simulink library "speedgoatlib_mscp"  (R2024b)
settings: Solver=VariableStepAuto  StartTime=0.0  StopTime=10.0  RelTol=1e-3
libraries: slrealtimeethercatlib x517, simulink x316, hdlsllib x168, $bdroot x11, slrealtimeutilitieslib x1
(part 2 of 5)

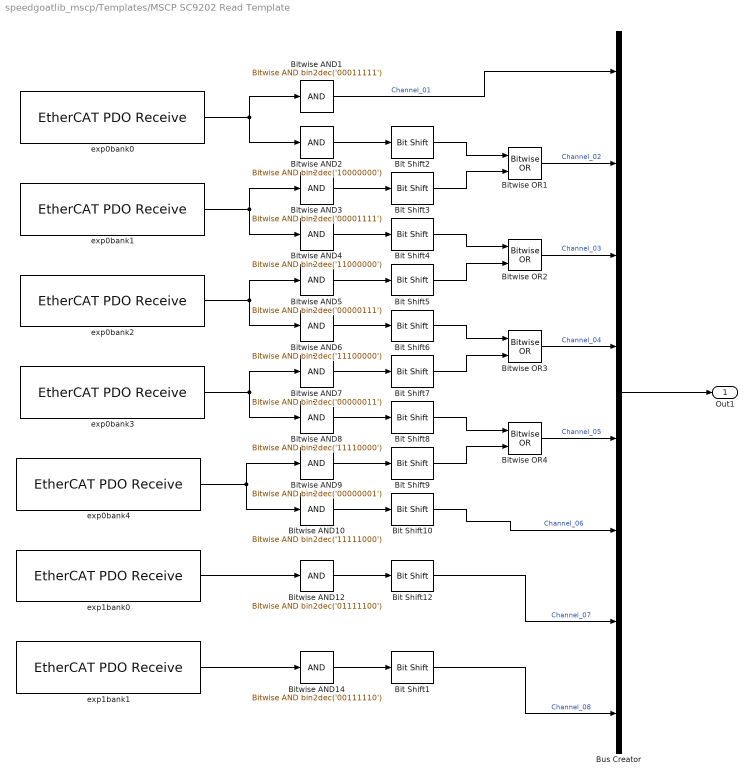
== system speedgoatlib_mscp/Templates/MSCP SC9202 Read Template ==
  Bit Shift1 : hdlsllib/Logic and Bit Operations/Bit Shift  mode=Shift Right Logical  N=1
  Bit Shift10 : hdlsllib/Logic and Bit Operations/Bit Shift  mode=Shift Right Logical  N=3
  Bit Shift12 : hdlsllib/Logic and Bit Operations/Bit Shift  mode=Shift Right Logical  N=2
  Bit Shift2 : hdlsllib/Logic and Bit Operations/Bit Shift  mode=Shift Right Logical  N=7
  Bit Shift3 : hdlsllib/Logic and Bit Operations/Bit Shift  mode=Shift Left Logical  N=1
  Bit Shift4 : hdlsllib/Logic and Bit Operations/Bit Shift  mode=Shift Right Logical  N=6
  Bit Shift5 : hdlsllib/Logic and Bit Operations/Bit Shift  mode=Shift Left Logical  N=2
  Bit Shift6 : hdlsllib/Logic and Bit Operations/Bit Shift  mode=Shift Right Logical  N=5
  Bit Shift7 : hdlsllib/Logic and Bit Operations/Bit Shift  mode=Shift Left Logical  N=3
  Bit Shift8 : hdlsllib/Logic and Bit Operations/Bit Shift  mode=Shift Right Logical  N=4
  Bit Shift9 : hdlsllib/Logic and Bit Operations/Bit Shift  mode=Shift Left Logical  N=4
  Bitwise AND1 : simulink/Logic and Bit Operations/Bitwise Operator  logicop=AND  UseBitMask=on  BitMask=bin2dec('00011111')  BitMaskRealWorld=Stored Integer
      settings: LibrarySourceBlock=|
      | simulink/Quick Insert/Logic and Bit
      | Operations/Bitwise AND
  Bitwise AND10 : simulink/Logic and Bit Operations/Bitwise Operator  logicop=AND  UseBitMask=on  BitMask=bin2dec('11111000')  BitMaskRealWorld=Stored Integer
      settings: LibrarySourceBlock=|
      | simulink/Quick Insert/Logic and Bit
      | Operations/Bitwise AND
  Bitwise AND12 : simulink/Logic and Bit Operations/Bitwise Operator  logicop=AND  UseBitMask=on  BitMask=bin2dec('01111100')  BitMaskRealWorld=Stored Integer
      settings: LibrarySourceBlock=|
      | simulink/Quick Insert/Logic and Bit
      | Operations/Bitwise AND
  Bitwise AND14 : simulink/Logic and Bit Operations/Bitwise Operator  logicop=AND  UseBitMask=on  BitMask=bin2dec('00111110')  BitMaskRealWorld=Stored Integer
      settings: LibrarySourceBlock=|
      | simulink/Quick Insert/Logic and Bit
      | Operations/Bitwise AND
  Bitwise AND2 : simulink/Logic and Bit Operations/Bitwise Operator  logicop=AND  UseBitMask=on  BitMask=bin2dec('10000000')  BitMaskRealWorld=Stored Integer
      settings: LibrarySourceBlock=|
      | simulink/Quick Insert/Logic and Bit
      | Operations/Bitwise AND
  Bitwise AND3 : simulink/Logic and Bit Operations/Bitwise Operator  logicop=AND  UseBitMask=on  BitMask=bin2dec('00001111')  BitMaskRealWorld=Stored Integer
      settings: LibrarySourceBlock=|
      | simulink/Quick Insert/Logic and Bit
      | Operations/Bitwise AND
  Bitwise AND4 : simulink/Logic and Bit Operations/Bitwise Operator  logicop=AND  UseBitMask=on  BitMask=bin2dec('11000000')  BitMaskRealWorld=Stored Integer
      settings: LibrarySourceBlock=|
      | simulink/Quick Insert/Logic and Bit
      | Operations/Bitwise AND
  Bitwise AND5 : simulink/Logic and Bit Operations/Bitwise Operator  logicop=AND  UseBitMask=on  BitMask=bin2dec('00000111')  BitMaskRealWorld=Stored Integer
      settings: LibrarySourceBlock=|
      | simulink/Quick Insert/Logic and Bit
      | Operations/Bitwise AND
  Bitwise AND6 : simulink/Logic and Bit Operations/Bitwise Operator  logicop=AND  UseBitMask=on  BitMask=bin2dec('11100000')  BitMaskRealWorld=Stored Integer
      settings: LibrarySourceBlock=|
      | simulink/Quick Insert/Logic and Bit
      | Operations/Bitwise AND
  Bitwise AND7 : simulink/Logic and Bit Operations/Bitwise Operator  logicop=AND  UseBitMask=on  BitMask=bin2dec('00000011')  BitMaskRealWorld=Stored Integer
      settings: LibrarySourceBlock=|
      | simulink/Quick Insert/Logic and Bit
      | Operations/Bitwise AND
  Bitwise AND8 : simulink/Logic and Bit Operations/Bitwise Operator  logicop=AND  UseBitMask=on  BitMask=bin2dec('11110000')  BitMaskRealWorld=Stored Integer
      settings: LibrarySourceBlock=|
      | simulink/Quick Insert/Logic and Bit
      | Operations/Bitwise AND
  Bitwise AND9 : simulink/Logic and Bit Operations/Bitwise Operator  logicop=AND  UseBitMask=on  BitMask=bin2dec('00000001')  BitMaskRealWorld=Stored Integer
      settings: LibrarySourceBlock=|
      | simulink/Quick Insert/Logic and Bit
      | Operations/Bitwise AND
  Bitwise OR{1..4} (4 alike) : simulink/Logic and Bit Operations/Bitwise Operator  logicop=OR  UseBitMask=off  NumInputPorts=2  BitMask=bin2dec('11011001')  BitMaskRealWorld=Stored Integer
      settings: LibrarySourceBlock=|
      | simulink/Quick Insert/Logic and Bit
      | Operations/Bitwise OR
  Bus Creator : BusCreator  Inputs=8  OutDataTypeStr=Bus: MscpBus_SC9202
      settings: InheritFromInputs=off
  exp0bank{0..4} (5 alike) : slrealtimeethercatlib/EtherCAT PDO Receive  Priority=2  sig_name=Uninitialized Block  sig_offset=144  sig_type=uint8  type_size=8  sig_dim=1  device_id=0  sample_time=0.010000
  exp1bank0 : slrealtimeethercatlib/EtherCAT PDO Receive  Priority=2  sig_name=Uninitialized Block  sig_offset=144  sig_type=uint8  type_size=8  sig_dim=1  device_id=0  sample_time=0.010000
  exp1bank1 : slrealtimeethercatlib/EtherCAT PDO Receive  Priority=2  sig_name=Uninitialized Block  sig_offset=144  sig_type=uint8  type_size=8  sig_dim=1  device_id=0  sample_time=0.010000
  Out1 : Outport
  wires:
  Bit Shift1/1 -> Bus Creator/8  "Channel_08"
  Bitwise AND14/1 -> Bit Shift1/1
  Bit Shift5/1 -> Bitwise OR2/2
  exp0bank3/1 -> Bitwise AND8/1, Bitwise AND7/1
  Bitwise OR2/1 -> Bus Creator/3  "Channel_03"
  exp1bank1/1 -> Bitwise AND14/1
  exp0bank4/1 -> Bitwise AND10/1, Bitwise AND9/1
  exp0bank0/1 -> Bitwise AND2/1, Bitwise AND1/1
  exp1bank0/1 -> Bitwise AND12/1
  exp0bank1/1 -> Bitwise AND3/1, Bitwise AND4/1
  Bitwise OR4/1 -> Bus Creator/5  "Channel_05"
  Bitwise AND8/1 -> Bit Shift8/1
  Bit Shift3/1 -> Bitwise OR1/2
  Bitwise AND12/1 -> Bit Shift12/1
  Bit Shift7/1 -> Bitwise OR3/2
  Bitwise AND6/1 -> Bit Shift6/1
  Bitwise OR1/1 -> Bus Creator/2  "Channel_02"
  exp0bank2/1 -> Bitwise AND5/1, Bitwise AND6/1
  Bit Shift8/1 -> Bitwise OR4/1
  Bit Shift12/1 -> Bus Creator/7  "Channel_07"
  Bit Shift9/1 -> Bitwise OR4/2
  Bit Shift2/1 -> Bitwise OR1/1
  Bitwise AND10/1 -> Bit Shift10/1
  Bitwise AND1/1 -> Bus Creator/1  "Channel_01"
  Bit Shift6/1 -> Bitwise OR3/1
  Bitwise AND4/1 -> Bit Shift4/1
  Bitwise OR3/1 -> Bus Creator/4  "Channel_04"
  Bit Shift10/1 -> Bus Creator/6  "Channel_06"
  Bus Creator/1 -> Out1/1
  Bitwise AND7/1 -> Bit Shift7/1
  Bitwise AND5/1 -> Bit Shift5/1
  Bitwise AND9/1 -> Bit Shift9/1
  Bitwise AND2/1 -> Bit Shift2/1
  Bit Shift4/1 -> Bitwise OR2/1
  Bitwise AND3/1 -> Bit Shift3/1

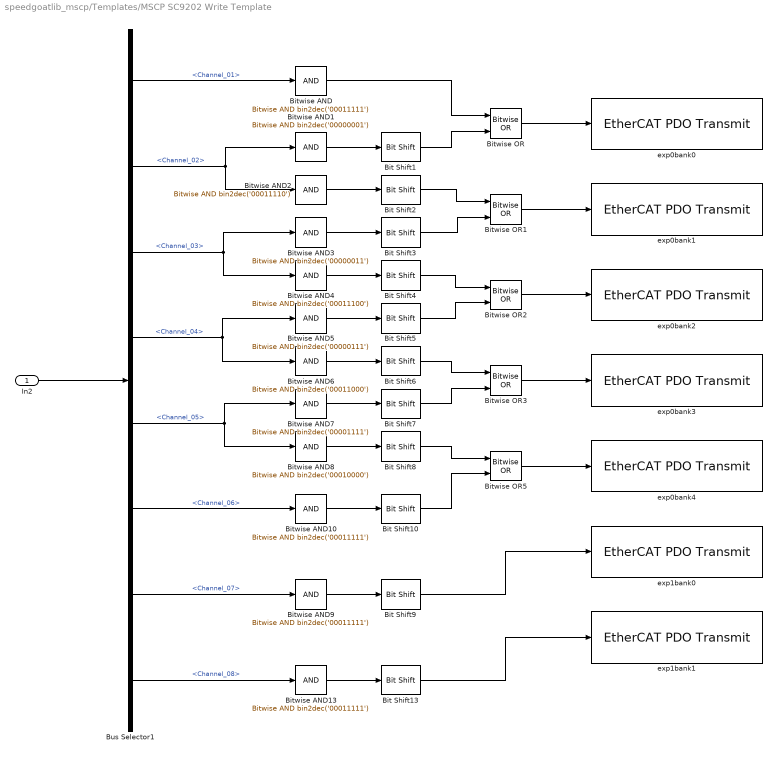
== system speedgoatlib_mscp/Templates/MSCP SC9202 Write Template ==
  In2 : Inport  OutDataTypeStr=Bus: MscpBus_SC9202
  Bit Shift1 : hdlsllib/Logic and Bit Operations/Bit Shift  mode=Shift Left Logical  N=7
  Bit Shift10 : hdlsllib/Logic and Bit Operations/Bit Shift  mode=Shift Left Logical  N=3
  Bit Shift13 : hdlsllib/Logic and Bit Operations/Bit Shift  mode=Shift Left Logical  N=1
  Bit Shift2 : hdlsllib/Logic and Bit Operations/Bit Shift  mode=Shift Right Logical  N=1
  Bit Shift3 : hdlsllib/Logic and Bit Operations/Bit Shift  mode=Shift Left Logical  N=6
  Bit Shift4 : hdlsllib/Logic and Bit Operations/Bit Shift  mode=Shift Right Logical  N=2
  Bit Shift5 : hdlsllib/Logic and Bit Operations/Bit Shift  mode=Shift Left Logical  N=5
  Bit Shift6 : hdlsllib/Logic and Bit Operations/Bit Shift  mode=Shift Right Logical  N=3
  Bit Shift7 : hdlsllib/Logic and Bit Operations/Bit Shift  mode=Shift Left Logical  N=4
  Bit Shift8 : hdlsllib/Logic and Bit Operations/Bit Shift  mode=Shift Right Logical  N=4
  Bit Shift9 : hdlsllib/Logic and Bit Operations/Bit Shift  mode=Shift Left Logical  N=2
  Bitwise AND{,9..10,13} (4 alike) : simulink/Logic and Bit Operations/Bitwise Operator  logicop=AND  UseBitMask=on  BitMask=bin2dec('00011111')  BitMaskRealWorld=Stored Integer
      settings: LibrarySourceBlock=|
      | simulink/Quick Insert/Logic and Bit
      | Operations/Bitwise AND
  Bitwise AND1 : simulink/Logic and Bit Operations/Bitwise Operator  logicop=AND  UseBitMask=on  BitMask=bin2dec('00000001')  BitMaskRealWorld=Stored Integer
      settings: LibrarySourceBlock=|
      | simulink/Quick Insert/Logic and Bit
      | Operations/Bitwise AND
  Bitwise AND2 : simulink/Logic and Bit Operations/Bitwise Operator  logicop=AND  UseBitMask=on  BitMask=bin2dec('00011110')  BitMaskRealWorld=Stored Integer
      settings: LibrarySourceBlock=|
      | simulink/Quick Insert/Logic and Bit
      | Operations/Bitwise AND
  Bitwise AND3 : simulink/Logic and Bit Operations/Bitwise Operator  logicop=AND  UseBitMask=on  BitMask=bin2dec('00000011')  BitMaskRealWorld=Stored Integer
      settings: LibrarySourceBlock=|
      | simulink/Quick Insert/Logic and Bit
      | Operations/Bitwise AND
  Bitwise AND4 : simulink/Logic and Bit Operations/Bitwise Operator  logicop=AND  UseBitMask=on  BitMask=bin2dec('00011100')  BitMaskRealWorld=Stored Integer
      settings: LibrarySourceBlock=|
      | simulink/Quick Insert/Logic and Bit
      | Operations/Bitwise AND
  Bitwise AND5 : simulink/Logic and Bit Operations/Bitwise Operator  logicop=AND  UseBitMask=on  BitMask=bin2dec('00000111')  BitMaskRealWorld=Stored Integer
      settings: LibrarySourceBlock=|
      | simulink/Quick Insert/Logic and Bit
      | Operations/Bitwise AND
  Bitwise AND6 : simulink/Logic and Bit Operations/Bitwise Operator  logicop=AND  UseBitMask=on  BitMask=bin2dec('00011000')  BitMaskRealWorld=Stored Integer
      settings: LibrarySourceBlock=|
      | simulink/Quick Insert/Logic and Bit
      | Operations/Bitwise AND
  Bitwise AND7 : simulink/Logic and Bit Operations/Bitwise Operator  logicop=AND  UseBitMask=on  BitMask=bin2dec('00001111')  BitMaskRealWorld=Stored Integer
      settings: LibrarySourceBlock=|
      | simulink/Quick Insert/Logic and Bit
      | Operations/Bitwise AND
  Bitwise AND8 : simulink/Logic and Bit Operations/Bitwise Operator  logicop=AND  UseBitMask=on  BitMask=bin2dec('00010000')  BitMaskRealWorld=Stored Integer
      settings: LibrarySourceBlock=|
      | simulink/Quick Insert/Logic and Bit
      | Operations/Bitwise AND
  Bitwise OR{,1..3,5} (5 alike) : simulink/Logic and Bit Operations/Bitwise Operator  logicop=OR  UseBitMask=off  NumInputPorts=2  BitMask=bin2dec('11011001')  BitMaskRealWorld=Stored Integer
      settings: LibrarySourceBlock=|
      | simulink/Quick Insert/Logic and Bit
      | Operations/Bitwise OR
  Bus Selector1 : BusSelector  OutputSignals=Channel_01,Channel_02,Channel_03,Channel_04,Channel_05,Channel_06,Channel_07,Channel_08
  exp0bank{0..4} (5 alike) : slrealtimeethercatlib/EtherCAT PDO Transmit  Priority=3  sig_name=Uninitialized Block  sig_offset=128  sig_type=uint8  type_size=8  sig_dim=1  device_id=0  sample_time=0.010000
  exp1bank0 : slrealtimeethercatlib/EtherCAT PDO Transmit  Priority=3  sig_name=Uninitialized Block  sig_offset=128  sig_type=uint8  type_size=8  sig_dim=1  device_id=0  sample_time=0.010000
  exp1bank1 : slrealtimeethercatlib/EtherCAT PDO Transmit  Priority=3  sig_name=Uninitialized Block  sig_offset=128  sig_type=uint8  type_size=8  sig_dim=1  device_id=0  sample_time=0.010000
  wires:
  Bus Selector1/2 -> Bitwise AND1/1, Bitwise AND2/1  "<Channel_02>"
  Bitwise AND6/1 -> Bit Shift6/1
  Bitwise AND3/1 -> Bit Shift3/1
  Bitwise OR/1 -> exp0bank0/1
  Bitwise AND4/1 -> Bit Shift4/1
  In2/1 -> Bus Selector1/1
  Bitwise AND5/1 -> Bit Shift5/1
  Bit Shift2/1 -> Bitwise OR1/1
  Bitwise AND1/1 -> Bit Shift1/1
  Bus Selector1/1 -> Bitwise AND/1  "<Channel_01>"
  Bit Shift1/1 -> Bitwise OR/2
  Bitwise AND2/1 -> Bit Shift2/1
  Bitwise AND10/1 -> Bit Shift10/1
  Bitwise AND/1 -> Bitwise OR/1
  Bit Shift3/1 -> Bitwise OR1/2
  Bitwise AND7/1 -> Bit Shift7/1
  Bitwise AND8/1 -> Bit Shift8/1
  Bitwise OR1/1 -> exp0bank1/1
  Bus Selector1/5 -> Bitwise AND8/1, Bitwise AND7/1  "<Channel_05>"
  Bus Selector1/3 -> Bitwise AND3/1, Bitwise AND4/1  "<Channel_03>"
  Bit Shift4/1 -> Bitwise OR2/1
  Bit Shift5/1 -> Bitwise OR2/2
  Bus Selector1/4 -> Bitwise AND5/1, Bitwise AND6/1  "<Channel_04>"
  Bitwise OR2/1 -> exp0bank2/1
  Bit Shift6/1 -> Bitwise OR3/1
  Bit Shift7/1 -> Bitwise OR3/2
  Bitwise OR3/1 -> exp0bank3/1
  Bit Shift8/1 -> Bitwise OR5/1
  Bit Shift10/1 -> Bitwise OR5/2
  Bitwise OR5/1 -> exp0bank4/1
  Bus Selector1/6 -> Bitwise AND10/1  "<Channel_06>"
  Bit Shift9/1 -> exp1bank0/1
  Bitwise AND9/1 -> Bit Shift9/1
  Bus Selector1/7 -> Bitwise AND9/1  "<Channel_07>"
  Bitwise AND13/1 -> Bit Shift13/1
  Bit Shift13/1 -> exp1bank1/1
  Bus Selector1/8 -> Bitwise AND13/1  "<Channel_08>"

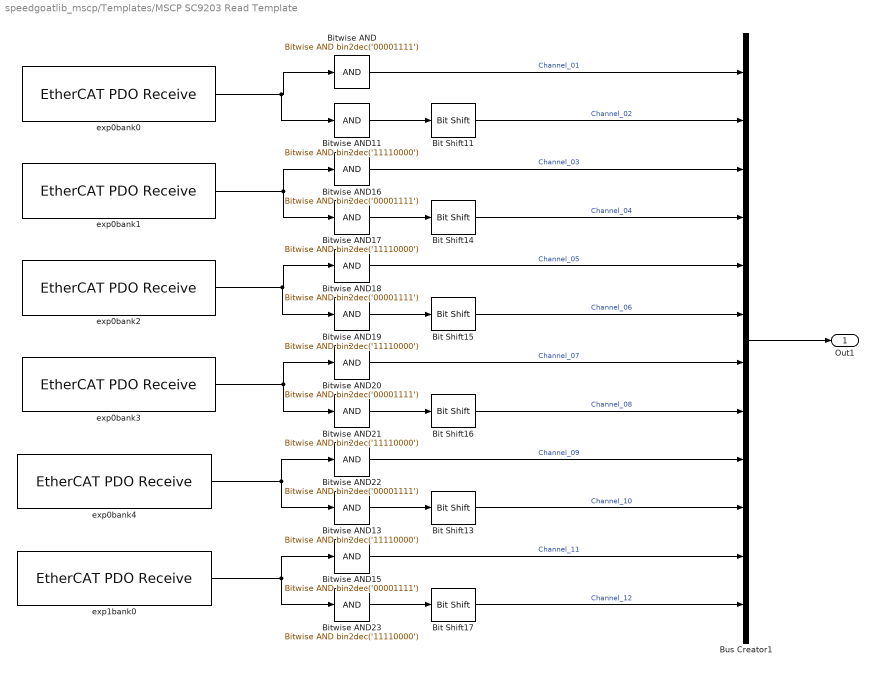
== system speedgoatlib_mscp/Templates/MSCP SC9203 Read Template ==
  Bit Shift{11,13..17} (6 alike) : hdlsllib/Logic and Bit Operations/Bit Shift  mode=Shift Right Logical  N=4
  Bitwise AND{,15..16,18,20,22} (6 alike) : simulink/Logic and Bit Operations/Bitwise Operator  logicop=AND  UseBitMask=on  BitMask=bin2dec('00001111')  BitMaskRealWorld=Stored Integer
      settings: LibrarySourceBlock=|
      | simulink/Quick Insert/Logic and Bit
      | Operations/Bitwise AND
  Bitwise AND{11,13,17,19,21,23} (6 alike) : simulink/Logic and Bit Operations/Bitwise Operator  logicop=AND  UseBitMask=on  BitMask=bin2dec('11110000')  BitMaskRealWorld=Stored Integer
      settings: LibrarySourceBlock=|
      | simulink/Quick Insert/Logic and Bit
      | Operations/Bitwise AND
  Bus Creator1 : BusCreator  Inputs=12  OutDataTypeStr=Bus: MscpBus_SC9203
      settings: InheritFromInputs=off
  exp0bank{0..4} (5 alike) : slrealtimeethercatlib/EtherCAT PDO Receive  Priority=2  sig_name=Uninitialized Block  sig_offset=144  sig_type=uint8  type_size=8  sig_dim=1  device_id=0  sample_time=0.010000
  exp1bank0 : slrealtimeethercatlib/EtherCAT PDO Receive  Priority=2  sig_name=Uninitialized Block  sig_offset=144  sig_type=uint8  type_size=8  sig_dim=1  device_id=0  sample_time=0.010000
  Out1 : Outport
  wires:
  Bitwise AND15/1 -> Bus Creator1/11  "Channel_11"
  Bitwise AND20/1 -> Bus Creator1/7  "Channel_07"
  Bitwise AND22/1 -> Bus Creator1/9  "Channel_09"
  Bitwise AND16/1 -> Bus Creator1/3  "Channel_03"
  Bit Shift17/1 -> Bus Creator1/12  "Channel_12"
  Bitwise AND23/1 -> Bit Shift17/1
  Bitwise AND19/1 -> Bit Shift15/1
  Bitwise AND/1 -> Bus Creator1/1  "Channel_01"
  Bitwise AND11/1 -> Bit Shift11/1
  Bit Shift15/1 -> Bus Creator1/6  "Channel_06"
  Bitwise AND13/1 -> Bit Shift13/1
  Bitwise AND21/1 -> Bit Shift16/1
  Bit Shift14/1 -> Bus Creator1/4  "Channel_04"
  Bit Shift11/1 -> Bus Creator1/2  "Channel_02"
  Bit Shift16/1 -> Bus Creator1/8  "Channel_08"
  Bitwise AND17/1 -> Bit Shift14/1
  Bitwise AND18/1 -> Bus Creator1/5  "Channel_05"
  Bit Shift13/1 -> Bus Creator1/10  "Channel_10"
  exp0bank0/1 -> Bitwise AND11/1, Bitwise AND/1
  exp0bank1/1 -> Bitwise AND17/1, Bitwise AND16/1
  exp0bank2/1 -> Bitwise AND19/1, Bitwise AND18/1
  exp0bank3/1 -> Bitwise AND21/1, Bitwise AND20/1
  exp0bank4/1 -> Bitwise AND13/1, Bitwise AND22/1
  exp1bank0/1 -> Bitwise AND23/1, Bitwise AND15/1
  Bus Creator1/1 -> Out1/1

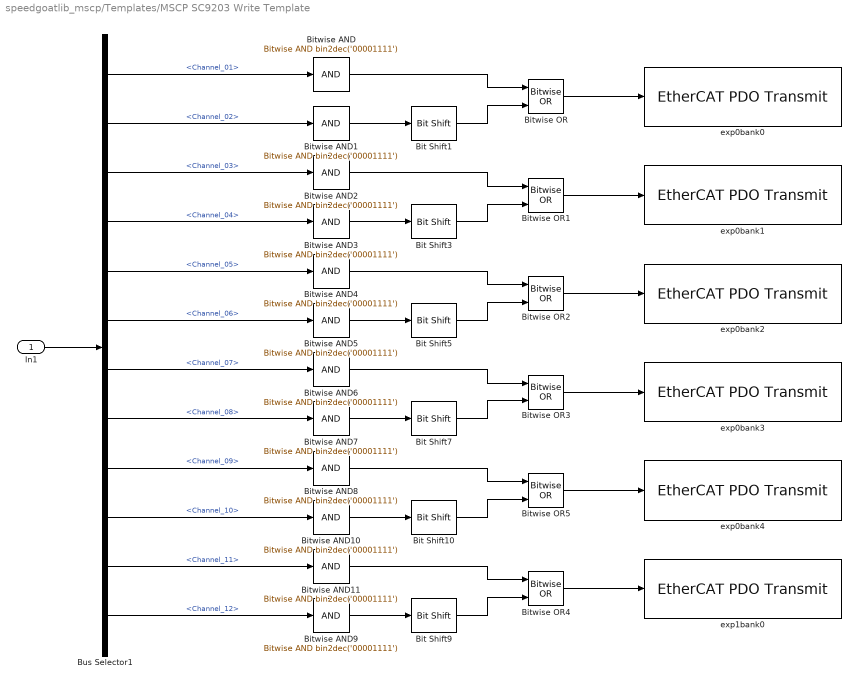
== system speedgoatlib_mscp/Templates/MSCP SC9203 Write Template ==
  In1 : Inport  OutDataTypeStr=Bus: MscpBus_SC9203
  Bit Shift{1,3,5,7,9..10} (6 alike) : hdlsllib/Logic and Bit Operations/Bit Shift  mode=Shift Left Logical  N=4
  Bitwise AND{,1..11} (12 alike) : simulink/Logic and Bit Operations/Bitwise Operator  logicop=AND  UseBitMask=on  BitMask=bin2dec('00001111')  BitMaskRealWorld=Stored Integer
      settings: LibrarySourceBlock=|
      | simulink/Quick Insert/Logic and Bit
      | Operations/Bitwise AND
  Bitwise OR{,1..5} (6 alike) : simulink/Logic and Bit Operations/Bitwise Operator  logicop=OR  UseBitMask=off  NumInputPorts=2  BitMask=bin2dec('11011001')  BitMaskRealWorld=Stored Integer
      settings: LibrarySourceBlock=|
      | simulink/Quick Insert/Logic and Bit
      | Operations/Bitwise OR
  Bus Selector1 : BusSelector  OutputSignals=Channel_01,Channel_02,Channel_03,Channel_04,Channel_05,Channel_06,Channel_07,Channel_08,Channel_09,Channel_10,Channel_11,Channel_12
  exp0bank{0..4} (5 alike) : slrealtimeethercatlib/EtherCAT PDO Transmit  Priority=3  sig_name=Uninitialized Block  sig_offset=128  sig_type=uint8  type_size=8  sig_dim=1  device_id=0  sample_time=0.010000
  exp1bank0 : slrealtimeethercatlib/EtherCAT PDO Transmit  Priority=3  sig_name=Uninitialized Block  sig_offset=128  sig_type=uint8  type_size=8  sig_dim=1  device_id=0  sample_time=0.010000
  wires:
  Bitwise AND6/1 -> Bitwise OR3/1
  Bit Shift7/1 -> Bitwise OR3/2
  Bitwise OR2/1 -> exp0bank2/1
  Bitwise OR3/1 -> exp0bank3/1
  Bit Shift3/1 -> Bitwise OR1/2
  Bit Shift1/1 -> Bitwise OR/2
  Bitwise OR1/1 -> exp0bank1/1
  Bus Selector1/1 -> Bitwise AND/1  "<Channel_01>"
  Bitwise AND8/1 -> Bitwise OR5/1
  Bitwise AND4/1 -> Bitwise OR2/1
  Bitwise AND7/1 -> Bit Shift7/1
  Bitwise AND10/1 -> Bit Shift10/1
  Bus Selector1/2 -> Bitwise AND1/1  "<Channel_02>"
  In1/1 -> Bus Selector1/1
  Bitwise AND3/1 -> Bit Shift3/1
  Bit Shift10/1 -> Bitwise OR5/2
  Bit Shift5/1 -> Bitwise OR2/2
  Bitwise AND1/1 -> Bit Shift1/1
  Bitwise OR/1 -> exp0bank0/1
  Bitwise AND5/1 -> Bit Shift5/1
  Bitwise AND/1 -> Bitwise OR/1
  Bitwise OR5/1 -> exp0bank4/1
  Bitwise AND2/1 -> Bitwise OR1/1
  Bitwise AND9/1 -> Bit Shift9/1
  Bus Selector1/3 -> Bitwise AND2/1  "<Channel_03>"
  Bus Selector1/4 -> Bitwise AND3/1  "<Channel_04>"
  Bus Selector1/5 -> Bitwise AND4/1  "<Channel_05>"
  Bus Selector1/6 -> Bitwise AND5/1  "<Channel_06>"
  Bus Selector1/7 -> Bitwise AND6/1  "<Channel_07>"
  Bus Selector1/8 -> Bitwise AND7/1  "<Channel_08>"
  Bus Selector1/9 -> Bitwise AND8/1  "<Channel_09>"
  Bus Selector1/10 -> Bitwise AND10/1  "<Channel_10>"
  Bitwise OR4/1 -> exp1bank0/1
  Bit Shift9/1 -> Bitwise OR4/2
  Bitwise AND11/1 -> Bitwise OR4/1
  Bus Selector1/11 -> Bitwise AND11/1  "<Channel_11>"
  Bus Selector1/12 -> Bitwise AND9/1  "<Channel_12>"

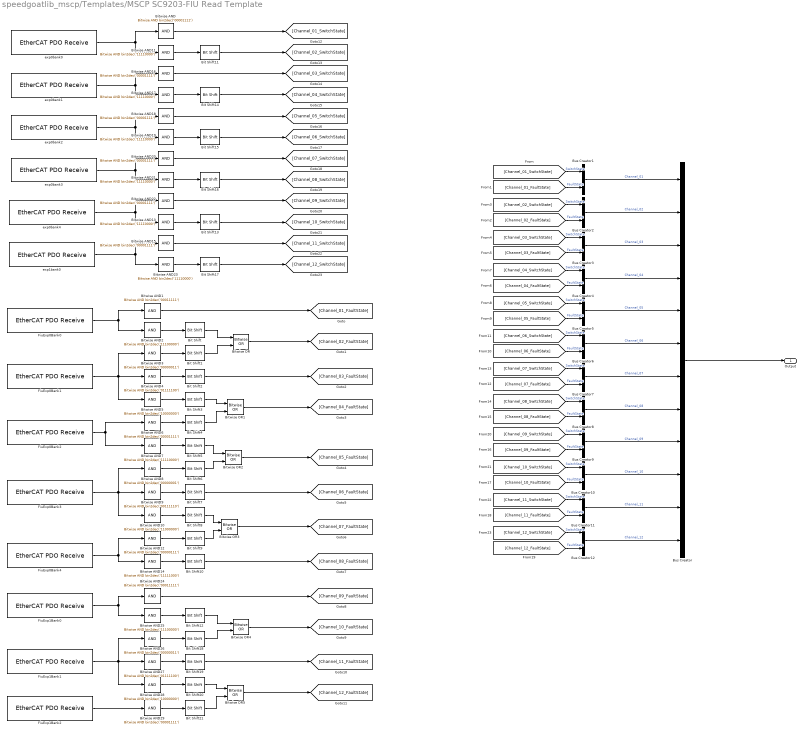
== system speedgoatlib_mscp/Templates/MSCP SC9203-FIU Read Template ==
  Bit Shift : hdlsllib/Logic and Bit Operations/Bit Shift  mode=Shift Right Logical  N=5
  Bit Shift1 : hdlsllib/Logic and Bit Operations/Bit Shift  mode=Shift Left Logical  N=3
  Bit Shift10 : hdlsllib/Logic and Bit Operations/Bit Shift  mode=Shift Right Logical  N=3
  Bit Shift{5,11,13..17} (7 alike) : hdlsllib/Logic and Bit Operations/Bit Shift  mode=Shift Right Logical  N=4
  Bit Shift12 : hdlsllib/Logic and Bit Operations/Bit Shift  mode=Shift Right Logical  N=5
  Bit Shift18 : hdlsllib/Logic and Bit Operations/Bit Shift  mode=Shift Left Logical  N=3
  Bit Shift19 : hdlsllib/Logic and Bit Operations/Bit Shift  mode=Shift Right Logical  N=2
  Bit Shift2 : hdlsllib/Logic and Bit Operations/Bit Shift  mode=Shift Right Logical  N=2
  Bit Shift20 : hdlsllib/Logic and Bit Operations/Bit Shift  mode=Shift Right Logical  N=7
  Bit Shift21 : hdlsllib/Logic and Bit Operations/Bit Shift  mode=Shift Left Logical  N=1
  Bit Shift3 : hdlsllib/Logic and Bit Operations/Bit Shift  mode=Shift Right Logical  N=7
  Bit Shift4 : hdlsllib/Logic and Bit Operations/Bit Shift  mode=Shift Left Logical  N=1
  Bit Shift6 : hdlsllib/Logic and Bit Operations/Bit Shift  mode=Shift Left Logical  N=4
  Bit Shift7 : hdlsllib/Logic and Bit Operations/Bit Shift  mode=Shift Right Logical  N=1
  Bit Shift8 : hdlsllib/Logic and Bit Operations/Bit Shift  mode=Shift Right Logical  N=6
  Bit Shift9 : hdlsllib/Logic and Bit Operations/Bit Shift  mode=Shift Left Logical  N=2
  Bitwise AND{,6,15..16,18,20,22,29} (8 alike) : simulink/Logic and Bit Operations/Bitwise Operator  logicop=AND  UseBitMask=on  BitMask=bin2dec('00001111')  BitMaskRealWorld=Stored Integer
      settings: LibrarySourceBlock=|
      | simulink/Quick Insert/Logic and Bit
      | Operations/Bitwise AND
  Bitwise AND1 : simulink/Logic and Bit Operations/Bitwise Operator  logicop=AND  UseBitMask=on  BitMask=bin2dec('00011111')  BitMaskRealWorld=Stored Integer
      settings: LibrarySourceBlock=|
      | simulink/Quick Insert/Logic and Bit
      | Operations/Bitwise AND
  Bitwise AND10 : simulink/Logic and Bit Operations/Bitwise Operator  logicop=AND  UseBitMask=on  BitMask=bin2dec('11000000')  BitMaskRealWorld=Stored Integer
      settings: LibrarySourceBlock=|
      | simulink/Quick Insert/Logic and Bit
      | Operations/Bitwise AND
  Bitwise AND{7,11,13,17,19,21,23} (7 alike) : simulink/Logic and Bit Operations/Bitwise Operator  logicop=AND  UseBitMask=on  BitMask=bin2dec('11110000')  BitMaskRealWorld=Stored Integer
      settings: LibrarySourceBlock=|
      | simulink/Quick Insert/Logic and Bit
      | Operations/Bitwise AND
  Bitwise AND12 : simulink/Logic and Bit Operations/Bitwise Operator  logicop=AND  UseBitMask=on  BitMask=bin2dec('00000111')  BitMaskRealWorld=Stored Integer
      settings: LibrarySourceBlock=|
      | simulink/Quick Insert/Logic and Bit
      | Operations/Bitwise AND
  Bitwise AND14 : simulink/Logic and Bit Operations/Bitwise Operator  logicop=AND  UseBitMask=on  BitMask=bin2dec('11111000')  BitMaskRealWorld=Stored Integer
      settings: LibrarySourceBlock=|
      | simulink/Quick Insert/Logic and Bit
      | Operations/Bitwise AND
  Bitwise AND2 : simulink/Logic and Bit Operations/Bitwise Operator  logicop=AND  UseBitMask=on  BitMask=bin2dec('11100000')  BitMaskRealWorld=Stored Integer
      settings: LibrarySourceBlock=|
      | simulink/Quick Insert/Logic and Bit
      | Operations/Bitwise AND
  Bitwise AND24 : simulink/Logic and Bit Operations/Bitwise Operator  logicop=AND  UseBitMask=on  BitMask=bin2dec('00011111')  BitMaskRealWorld=Stored Integer
      settings: LibrarySourceBlock=|
      | simulink/Quick Insert/Logic and Bit
      | Operations/Bitwise AND
  Bitwise AND25 : simulink/Logic and Bit Operations/Bitwise Operator  logicop=AND  UseBitMask=on  BitMask=bin2dec('11100000')  BitMaskRealWorld=Stored Integer
      settings: LibrarySourceBlock=|
      | simulink/Quick Insert/Logic and Bit
      | Operations/Bitwise AND
  Bitwise AND26 : simulink/Logic and Bit Operations/Bitwise Operator  logicop=AND  UseBitMask=on  BitMask=bin2dec('00000011')  BitMaskRealWorld=Stored Integer
      settings: LibrarySourceBlock=|
      | simulink/Quick Insert/Logic and Bit
      | Operations/Bitwise AND
  Bitwise AND27 : simulink/Logic and Bit Operations/Bitwise Operator  logicop=AND  UseBitMask=on  BitMask=bin2dec('01111100')  BitMaskRealWorld=Stored Integer
      settings: LibrarySourceBlock=|
      | simulink/Quick Insert/Logic and Bit
      | Operations/Bitwise AND
  Bitwise AND28 : simulink/Logic and Bit Operations/Bitwise Operator  logicop=AND  UseBitMask=on  BitMask=bin2dec('10000000')  BitMaskRealWorld=Stored Integer
      settings: LibrarySourceBlock=|
      | simulink/Quick Insert/Logic and Bit
      | Operations/Bitwise AND
  Bitwise AND3 : simulink/Logic and Bit Operations/Bitwise Operator  logicop=AND  UseBitMask=on  BitMask=bin2dec('00000011')  BitMaskRealWorld=Stored Integer
      settings: LibrarySourceBlock=|
      | simulink/Quick Insert/Logic and Bit
      | Operations/Bitwise AND
  Bitwise AND4 : simulink/Logic and Bit Operations/Bitwise Operator  logicop=AND  UseBitMask=on  BitMask=bin2dec('01111100')  BitMaskRealWorld=Stored Integer
      settings: LibrarySourceBlock=|
      | simulink/Quick Insert/Logic and Bit
      | Operations/Bitwise AND
  Bitwise AND5 : simulink/Logic and Bit Operations/Bitwise Operator  logicop=AND  UseBitMask=on  BitMask=bin2dec('10000000')  BitMaskRealWorld=Stored Integer
      settings: LibrarySourceBlock=|
      | simulink/Quick Insert/Logic and Bit
      | Operations/Bitwise AND
  Bitwise AND8 : simulink/Logic and Bit Operations/Bitwise Operator  logicop=AND  UseBitMask=on  BitMask=bin2dec('00000001')  BitMaskRealWorld=Stored Integer
      settings: LibrarySourceBlock=|
      | simulink/Quick Insert/Logic and Bit
      | Operations/Bitwise AND
  Bitwise AND9 : simulink/Logic and Bit Operations/Bitwise Operator  logicop=AND  UseBitMask=on  BitMask=bin2dec('00111110')  BitMaskRealWorld=Stored Integer
      settings: LibrarySourceBlock=|
      | simulink/Quick Insert/Logic and Bit
      | Operations/Bitwise AND
  Bitwise OR{,1..5} (6 alike) : simulink/Logic and Bit Operations/Bitwise Operator  logicop=OR  UseBitMask=off  NumInputPorts=2  BitMask=bin2dec('11011001')  BitMaskRealWorld=Stored Integer
      settings: LibrarySourceBlock=|
      | simulink/Quick Insert/Logic and Bit
      | Operations/Bitwise OR
  Bus Creator : BusCreator  Inputs=12  OutDataTypeStr=Bus: MscpBus_SC9203_FIU
      settings: InheritFromInputs=off
  Bus Creator{1..12} (12 alike) : BusCreator  Inputs=2  OutDataTypeStr=Bus: MscpBus_SC9203_FIU_Channel
      settings: InheritFromInputs=off
  FiuExp0Bank{0..4} (5 alike) : slrealtimeethercatlib/EtherCAT PDO Receive  Priority=2  sig_name=Uninitialized Block  sig_offset=144  sig_type=uint8  type_size=8  sig_dim=1  device_id=0  sample_time=0.010000
  FiuExp1Bank0 : slrealtimeethercatlib/EtherCAT PDO Receive  Priority=2  sig_name=Uninitialized Block  sig_offset=144  sig_type=uint8  type_size=8  sig_dim=1  device_id=0  sample_time=0.010000
  FiuExp1Bank1 : slrealtimeethercatlib/EtherCAT PDO Receive  Priority=2  sig_name=Uninitialized Block  sig_offset=144  sig_type=uint8  type_size=8  sig_dim=1  device_id=0  sample_time=0.010000
  FiuExp1Bank2 : slrealtimeethercatlib/EtherCAT PDO Receive  Priority=2  sig_name=Uninitialized Block  sig_offset=144  sig_type=uint8  type_size=8  sig_dim=1  device_id=0  sample_time=0.010000
  exp0bank{0..4} (5 alike) : slrealtimeethercatlib/EtherCAT PDO Receive  Priority=2  sig_name=Uninitialized Block  sig_offset=144  sig_type=uint8  type_size=8  sig_dim=1  device_id=0  sample_time=0.010000
  exp1bank0 : slrealtimeethercatlib/EtherCAT PDO Receive  Priority=2  sig_name=Uninitialized Block  sig_offset=144  sig_type=uint8  type_size=8  sig_dim=1  device_id=0  sample_time=0.010000
  Output : Outport
  wires:
  exp1bank0/1 -> Bitwise AND15/1, Bitwise AND23/1
  exp0bank4/1 -> Bitwise AND22/1, Bitwise AND13/1
  exp0bank3/1 -> Bitwise AND20/1, Bitwise AND21/1
  exp0bank2/1 -> Bitwise AND18/1, Bitwise AND19/1
  exp0bank1/1 -> Bitwise AND16/1, Bitwise AND17/1
  exp0bank0/1 -> Bitwise AND/1, Bitwise AND11/1
  Bitwise AND17/1 -> Bit Shift14/1
  Bitwise AND21/1 -> Bit Shift16/1
  Bitwise AND13/1 -> Bit Shift13/1
  Bitwise AND11/1 -> Bit Shift11/1
  Bitwise AND19/1 -> Bit Shift15/1
  Bitwise AND23/1 -> Bit Shift17/1
  Bitwise AND/1 -> [Channel_01_SwitchState]
  Bit Shift11/1 -> [Channel_02_SwitchState]
  Bitwise AND16/1 -> [Channel_03_SwitchState]
  Bit Shift14/1 -> [Channel_04_SwitchState]
  Bitwise AND18/1 -> [Channel_05_SwitchState]
  Bit Shift15/1 -> [Channel_06_SwitchState]
  Bitwise AND20/1 -> [Channel_07_SwitchState]
  Bit Shift16/1 -> [Channel_08_SwitchState]
  Bitwise AND22/1 -> [Channel_09_SwitchState]
  Bit Shift13/1 -> [Channel_10_SwitchState]
  Bitwise AND15/1 -> [Channel_11_SwitchState]
  Bit Shift17/1 -> [Channel_12_SwitchState]
  FiuExp0Bank0/1 -> Bitwise AND2/1, Bitwise AND1/1
  Bitwise AND1/1 -> [Channel_01_FaultState]
  Bit Shift1/1 -> Bitwise OR/2
  Bit Shift/1 -> Bitwise OR/1
  Bitwise OR/1 -> [Channel_02_FaultState]
  Bitwise AND3/1 -> Bit Shift1/1
  Bitwise AND2/1 -> Bit Shift/1
  FiuExp0Bank1/1 -> Bitwise AND3/1, Bitwise AND5/1, Bitwise AND4/1
  Bitwise AND4/1 -> Bit Shift2/1
  Bit Shift2/1 -> [Channel_03_FaultState]
  Bitwise AND5/1 -> Bit Shift3/1
  Bit Shift3/1 -> Bitwise OR1/1
  FiuExp0Bank2/1 -> Bitwise AND6/1, Bitwise AND7/1
  Bitwise AND6/1 -> Bit Shift4/1
  Bit Shift4/1 -> Bitwise OR1/2
  Bitwise OR1/1 -> [Channel_04_FaultState]
  Bitwise AND7/1 -> Bit Shift5/1
  Bit Shift5/1 -> Bitwise OR2/1
  Bit Shift6/1 -> Bitwise OR2/2
  Bitwise AND8/1 -> Bit Shift6/1
  FiuExp0Bank3/1 -> Bitwise AND10/1, Bitwise AND9/1, Bitwise AND8/1
  Bitwise OR2/1 -> [Channel_05_FaultState]
  Bitwise AND9/1 -> Bit Shift7/1
  Bit Shift7/1 -> [Channel_06_FaultState]
  Bitwise AND10/1 -> Bit Shift8/1
  FiuExp0Bank4/1 -> Bitwise AND14/1, Bitwise AND12/1
  Bitwise AND12/1 -> Bit Shift9/1
  Bit Shift8/1 -> Bitwise OR3/1
  Bit Shift9/1 -> Bitwise OR3/2
  Bitwise OR3/1 -> [Channel_07_FaultState]
  Bitwise AND14/1 -> Bit Shift10/1
  Bit Shift10/1 -> [Channel_08_FaultState]
  Bitwise OR5/1 -> [Channel_12_FaultState]
  Bit Shift21/1 -> Bitwise OR5/2
  Bitwise AND29/1 -> Bit Shift21/1
  FiuExp1Bank2/1 -> Bitwise AND29/1
  Bit Shift20/1 -> Bitwise OR5/1
  Bitwise AND28/1 -> Bit Shift20/1
  Bit Shift19/1 -> [Channel_11_FaultState]
  Bitwise AND27/1 -> Bit Shift19/1
  FiuExp1Bank1/1 -> Bitwise AND27/1, Bitwise AND28/1, Bitwise AND26/1
  Bitwise AND25/1 -> Bit Shift12/1
  Bitwise AND26/1 -> Bit Shift18/1
  Bitwise OR4/1 -> [Channel_10_FaultState]
  Bit Shift12/1 -> Bitwise OR4/1
  Bit Shift18/1 -> Bitwise OR4/2
  Bitwise AND24/1 -> [Channel_09_FaultState]
  FiuExp1Bank0/1 -> Bitwise AND24/1, Bitwise AND25/1
  Bus Creator/1 -> Output/1
  [Channel_01_SwitchState] -> Bus Creator1/1  "SwitchState"
  Bus Creator1/1 -> Bus Creator/1  "Channel_01"
  [Channel_01_FaultState] -> Bus Creator1/2  "FaultState"
  Bus Creator2/1 -> Bus Creator/2  "Channel_02"
  Bus Creator3/1 -> Bus Creator/3  "Channel_03"
  [Channel_02_SwitchState] -> Bus Creator2/1  "SwitchState"
  [Channel_02_FaultState] -> Bus Creator2/2  "FaultState"
  [Channel_03_SwitchState] -> Bus Creator3/1  "SwitchState"
  [Channel_03_FaultState] -> Bus Creator3/2  "FaultState"
  Bus Creator4/1 -> Bus Creator/4  "Channel_04"
  Bus Creator5/1 -> Bus Creator/5  "Channel_05"
  Bus Creator6/1 -> Bus Creator/6  "Channel_06"
  Bus Creator7/1 -> Bus Creator/7  "Channel_07"
  [Channel_04_SwitchState] -> Bus Creator4/1  "SwitchState"
  [Channel_04_FaultState] -> Bus Creator4/2  "FaultState"
  [Channel_05_SwitchState] -> Bus Creator5/1  "SwitchState"
  [Channel_05_FaultState] -> Bus Creator5/2  "FaultState"
  [Channel_07_SwitchState] -> Bus Creator7/1  "SwitchState"
  [Channel_07_FaultState] -> Bus Creator7/2  "FaultState"
  [Channel_06_FaultState] -> Bus Creator6/2  "FaultState"
  [Channel_06_SwitchState] -> Bus Creator6/1  "SwitchState"
  Bus Creator12/1 -> Bus Creator/12  "Channel_12"
  Bus Creator11/1 -> Bus Creator/11  "Channel_11"
  Bus Creator10/1 -> Bus Creator/10  "Channel_10"
  Bus Creator9/1 -> Bus Creator/9  "Channel_09"
  Bus Creator8/1 -> Bus Creator/8  "Channel_08"
  [Channel_08_SwitchState] -> Bus Creator8/1  "SwitchState"
  [Channel_08_FaultState] -> Bus Creator8/2  "FaultState"
  [Channel_09_SwitchState] -> Bus Creator9/1  "SwitchState"
  [Channel_09_FaultState] -> Bus Creator9/2  "FaultState"
  [Channel_10_SwitchState] -> Bus Creator10/1  "SwitchState"
  [Channel_10_FaultState] -> Bus Creator10/2  "FaultState"
  [Channel_11_SwitchState] -> Bus Creator11/1  "SwitchState"
  [Channel_11_FaultState] -> Bus Creator11/2  "FaultState"
  [Channel_12_SwitchState] -> Bus Creator12/1  "SwitchState"
  [Channel_12_FaultState] -> Bus Creator12/2  "FaultState"

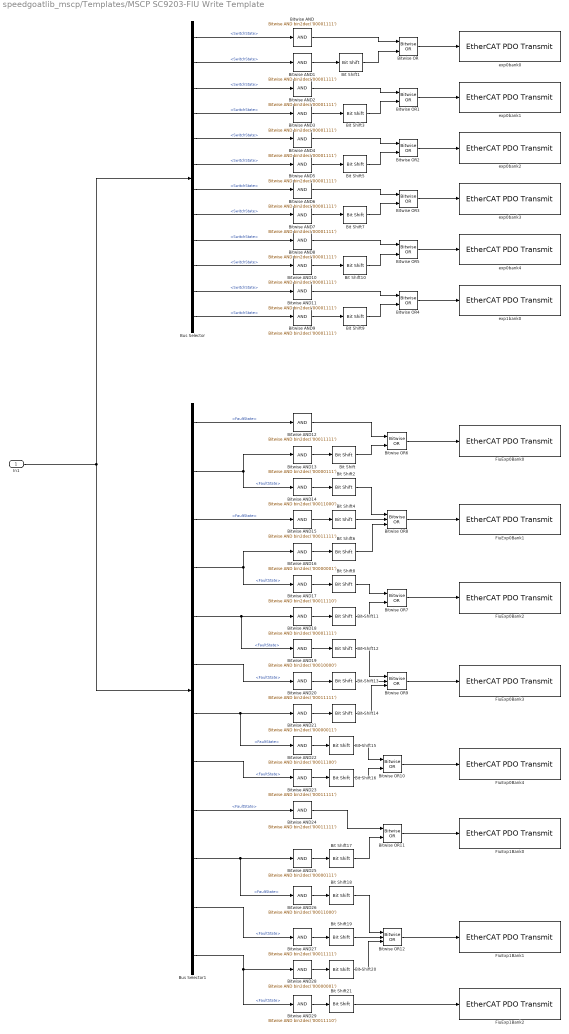
== system speedgoatlib_mscp/Templates/MSCP SC9203-FIU Write Template ==
  In1 : Inport  OutDataTypeStr=Bus: MscpBus_SC9203_FIU
  Bit Shift : hdlsllib/Logic and Bit Operations/Bit Shift  mode=Shift Left Logical  N=5
  Bit Shift{1,3,5,7,9..11} (7 alike) : hdlsllib/Logic and Bit Operations/Bit Shift  mode=Shift Left Logical  N=4
  Bit Shift12 : hdlsllib/Logic and Bit Operations/Bit Shift  mode=Shift Right Logical  N=4
  Bit Shift13 : hdlsllib/Logic and Bit Operations/Bit Shift  mode=Shift Left Logical  N=1
  Bit Shift14 : hdlsllib/Logic and Bit Operations/Bit Shift  mode=Shift Left Logical  N=6
  Bit Shift15 : hdlsllib/Logic and Bit Operations/Bit Shift  mode=Shift Right Logical  N=2
  Bit Shift16 : hdlsllib/Logic and Bit Operations/Bit Shift  mode=Shift Left Logical  N=3
  Bit Shift17 : hdlsllib/Logic and Bit Operations/Bit Shift  mode=Shift Left Logical  N=5
  Bit Shift18 : hdlsllib/Logic and Bit Operations/Bit Shift  mode=Shift Right Logical  N=3
  Bit Shift19 : hdlsllib/Logic and Bit Operations/Bit Shift  mode=Shift Left Logical  N=2
  Bit Shift2 : hdlsllib/Logic and Bit Operations/Bit Shift  mode=Shift Right Logical  N=3
  Bit Shift20 : hdlsllib/Logic and Bit Operations/Bit Shift  mode=Shift Left Logical  N=7
  Bit Shift21 : hdlsllib/Logic and Bit Operations/Bit Shift  mode=Shift Right Logical  N=1
  Bit Shift4 : hdlsllib/Logic and Bit Operations/Bit Shift  mode=Shift Left Logical  N=2
  Bit Shift6 : hdlsllib/Logic and Bit Operations/Bit Shift  mode=Shift Left Logical  N=7
  Bit Shift8 : hdlsllib/Logic and Bit Operations/Bit Shift  mode=Shift Right Logical  N=1
  Bitwise AND{,1..11,18} (13 alike) : simulink/Logic and Bit Operations/Bitwise Operator  logicop=AND  UseBitMask=on  BitMask=bin2dec('00001111')  BitMaskRealWorld=Stored Integer
      settings: LibrarySourceBlock=|
      | simulink/Quick Insert/Logic and Bit
      | Operations/Bitwise AND
  Bitwise AND{12,15,20,23..24,27} (6 alike) : simulink/Logic and Bit Operations/Bitwise Operator  logicop=AND  UseBitMask=on  BitMask=bin2dec('00011111')  BitMaskRealWorld=Stored Integer
      settings: LibrarySourceBlock=|
      | simulink/Quick Insert/Logic and Bit
      | Operations/Bitwise AND
  Bitwise AND13 : simulink/Logic and Bit Operations/Bitwise Operator  logicop=AND  UseBitMask=on  BitMask=bin2dec('00000111')  BitMaskRealWorld=Stored Integer
      settings: LibrarySourceBlock=|
      | simulink/Quick Insert/Logic and Bit
      | Operations/Bitwise AND
  Bitwise AND14 : simulink/Logic and Bit Operations/Bitwise Operator  logicop=AND  UseBitMask=on  BitMask=bin2dec('00011000')  BitMaskRealWorld=Stored Integer
      settings: LibrarySourceBlock=|
      | simulink/Quick Insert/Logic and Bit
      | Operations/Bitwise AND
  Bitwise AND16 : simulink/Logic and Bit Operations/Bitwise Operator  logicop=AND  UseBitMask=on  BitMask=bin2dec('00000001')  BitMaskRealWorld=Stored Integer
      settings: LibrarySourceBlock=|
      | simulink/Quick Insert/Logic and Bit
      | Operations/Bitwise AND
  Bitwise AND17 : simulink/Logic and Bit Operations/Bitwise Operator  logicop=AND  UseBitMask=on  BitMask=bin2dec('00011110')  BitMaskRealWorld=Stored Integer
      settings: LibrarySourceBlock=|
      | simulink/Quick Insert/Logic and Bit
      | Operations/Bitwise AND
  Bitwise AND19 : simulink/Logic and Bit Operations/Bitwise Operator  logicop=AND  UseBitMask=on  BitMask=bin2dec('00010000')  BitMaskRealWorld=Stored Integer
      settings: LibrarySourceBlock=|
      | simulink/Quick Insert/Logic and Bit
      | Operations/Bitwise AND
  Bitwise AND21 : simulink/Logic and Bit Operations/Bitwise Operator  logicop=AND  UseBitMask=on  BitMask=bin2dec('00000011')  BitMaskRealWorld=Stored Integer
      settings: LibrarySourceBlock=|
      | simulink/Quick Insert/Logic and Bit
      | Operations/Bitwise AND
  Bitwise AND22 : simulink/Logic and Bit Operations/Bitwise Operator  logicop=AND  UseBitMask=on  BitMask=bin2dec('00011100')  BitMaskRealWorld=Stored Integer
      settings: LibrarySourceBlock=|
      | simulink/Quick Insert/Logic and Bit
      | Operations/Bitwise AND
  Bitwise AND25 : simulink/Logic and Bit Operations/Bitwise Operator  logicop=AND  UseBitMask=on  BitMask=bin2dec('00000111')  BitMaskRealWorld=Stored Integer
      settings: LibrarySourceBlock=|
      | simulink/Quick Insert/Logic and Bit
      | Operations/Bitwise AND
  Bitwise AND26 : simulink/Logic and Bit Operations/Bitwise Operator  logicop=AND  UseBitMask=on  BitMask=bin2dec('00011000')  BitMaskRealWorld=Stored Integer
      settings: LibrarySourceBlock=|
      | simulink/Quick Insert/Logic and Bit
      | Operations/Bitwise AND
  Bitwise AND28 : simulink/Logic and Bit Operations/Bitwise Operator  logicop=AND  UseBitMask=on  BitMask=bin2dec('00000001')  BitMaskRealWorld=Stored Integer
      settings: LibrarySourceBlock=|
      | simulink/Quick Insert/Logic and Bit
      | Operations/Bitwise AND
  Bitwise AND29 : simulink/Logic and Bit Operations/Bitwise Operator  logicop=AND  UseBitMask=on  BitMask=bin2dec('00011110')  BitMaskRealWorld=Stored Integer
      settings: LibrarySourceBlock=|
      | simulink/Quick Insert/Logic and Bit
      | Operations/Bitwise AND
  Bitwise OR{,1..7,10..11} (10 alike) : simulink/Logic and Bit Operations/Bitwise Operator  logicop=OR  UseBitMask=off  NumInputPorts=2  BitMask=bin2dec('11011001')  BitMaskRealWorld=Stored Integer
      settings: LibrarySourceBlock=|
      | simulink/Quick Insert/Logic and Bit
      | Operations/Bitwise OR
  Bitwise OR12 : simulink/Logic and Bit Operations/Bitwise Operator  logicop=OR  UseBitMask=off  NumInputPorts=3  BitMask=bin2dec('11011001')  BitMaskRealWorld=Stored Integer
      settings: LibrarySourceBlock=|
      | simulink/Quick Insert/Logic and Bit
      | Operations/Bitwise OR
  Bitwise OR8 : simulink/Logic and Bit Operations/Bitwise Operator  logicop=OR  UseBitMask=off  NumInputPorts=3  BitMask=bin2dec('11011001')  BitMaskRealWorld=Stored Integer
      settings: LibrarySourceBlock=|
      | simulink/Quick Insert/Logic and Bit
      | Operations/Bitwise OR
  Bitwise OR9 : simulink/Logic and Bit Operations/Bitwise Operator  logicop=OR  UseBitMask=off  NumInputPorts=3  BitMask=bin2dec('11011001')  BitMaskRealWorld=Stored Integer
      settings: LibrarySourceBlock=|
      | simulink/Quick Insert/Logic and Bit
      | Operations/Bitwise OR
  Bus Selector : BusSelector  OutputSignals=Channel_01.SwitchState,Channel_02.SwitchState,Channel_03.SwitchState,Channel_04.SwitchState,Channel_05.SwitchState,Channel_06.SwitchState,Channel_07.SwitchState,Channel_08.SwitchState,Channel_09.SwitchState,Channel_10.SwitchState,Channel_11.SwitchState,Channel_12.SwitchState
  Bus Selector1 : BusSelector  OutputSignals=Channel_01.FaultState,Channel_02.FaultState,Channel_03.FaultState,Channel_04.FaultState,Channel_05.FaultState,Channel_06.FaultState,Channel_07.FaultState,Channel_08.FaultState,Channel_09.FaultState,Channel_10.FaultState,Channel_11.FaultState,Channel_12.FaultState
  FiuExp0Bank{0..4} (5 alike) : slrealtimeethercatlib/EtherCAT PDO Transmit  Priority=3  sig_name=Uninitialized Block  sig_offset=128  sig_type=uint8  type_size=8  sig_dim=1  device_id=0  sample_time=0.010000
  FiuExp1Bank0 : slrealtimeethercatlib/EtherCAT PDO Transmit  Priority=3  sig_name=Uninitialized Block  sig_offset=128  sig_type=uint8  type_size=8  sig_dim=1  device_id=0  sample_time=0.010000
  FiuExp1Bank1 : slrealtimeethercatlib/EtherCAT PDO Transmit  Priority=3  sig_name=Uninitialized Block  sig_offset=128  sig_type=uint8  type_size=8  sig_dim=1  device_id=0  sample_time=0.010000
  FiuExp1Bank2 : slrealtimeethercatlib/EtherCAT PDO Transmit  Priority=3  sig_name=Uninitialized Block  sig_offset=128  sig_type=uint8  type_size=8  sig_dim=1  device_id=0  sample_time=0.010000
  exp0bank{0..4} (5 alike) : slrealtimeethercatlib/EtherCAT PDO Transmit  Priority=3  sig_name=Uninitialized Block  sig_offset=128  sig_type=uint8  type_size=8  sig_dim=1  device_id=0  sample_time=0.010000
  exp1bank0 : slrealtimeethercatlib/EtherCAT PDO Transmit  Priority=3  sig_name=Uninitialized Block  sig_offset=128  sig_type=uint8  type_size=8  sig_dim=1  device_id=0  sample_time=0.010000
  wires:
  In1/1 -> Bus Selector1/1, Bus Selector/1
  Bus Selector/12 -> Bitwise AND9/1  "<SwitchState>"
  Bus Selector/11 -> Bitwise AND11/1  "<SwitchState>"
  Bitwise AND11/1 -> Bitwise OR4/1
  Bit Shift9/1 -> Bitwise OR4/2
  Bitwise OR4/1 -> exp1bank0/1
  Bus Selector/10 -> Bitwise AND10/1  "<SwitchState>"
  Bus Selector/9 -> Bitwise AND8/1  "<SwitchState>"
  Bus Selector/8 -> Bitwise AND7/1  "<SwitchState>"
  Bus Selector/7 -> Bitwise AND6/1  "<SwitchState>"
  Bus Selector/6 -> Bitwise AND5/1  "<SwitchState>"
  Bus Selector/4 -> Bitwise AND3/1  "<SwitchState>"
  Bitwise AND9/1 -> Bit Shift9/1
  Bitwise AND2/1 -> Bitwise OR1/1
  Bitwise OR5/1 -> exp0bank4/1
  Bitwise AND/1 -> Bitwise OR/1
  Bitwise AND5/1 -> Bit Shift5/1
  Bitwise OR/1 -> exp0bank0/1
  Bitwise AND1/1 -> Bit Shift1/1
  Bit Shift5/1 -> Bitwise OR2/2
  Bit Shift10/1 -> Bitwise OR5/2
  Bitwise AND3/1 -> Bit Shift3/1
  Bus Selector/2 -> Bitwise AND1/1  "<SwitchState>"
  Bitwise AND10/1 -> Bit Shift10/1
  Bitwise AND7/1 -> Bit Shift7/1
  Bitwise AND4/1 -> Bitwise OR2/1
  Bitwise AND8/1 -> Bitwise OR5/1
  Bus Selector/1 -> Bitwise AND/1  "<SwitchState>"
  Bitwise OR1/1 -> exp0bank1/1
  Bit Shift1/1 -> Bitwise OR/2
  Bit Shift3/1 -> Bitwise OR1/2
  Bitwise OR3/1 -> exp0bank3/1
  Bitwise OR2/1 -> exp0bank2/1
  Bit Shift7/1 -> Bitwise OR3/2
  Bitwise AND6/1 -> Bitwise OR3/1
  Bus Selector/3 -> Bitwise AND2/1  "<SwitchState>"
  Bus Selector/5 -> Bitwise AND4/1  "<SwitchState>"
  Bus Selector1/1 -> Bitwise AND12/1  "<FaultState>"
  Bitwise OR6/1 -> FiuExp0Bank0/1
  Bitwise AND13/1 -> Bit Shift/1
  Bit Shift/1 -> Bitwise OR6/2
  Bitwise AND12/1 -> Bitwise OR6/1
  Bus Selector1/2 -> Bitwise AND13/1, Bitwise AND14/1  "<FaultState>"
  Bit Shift2/1 -> Bitwise OR8/1
  Bit Shift4/1 -> Bitwise OR8/2
  Bitwise OR8/1 -> FiuExp0Bank1/1
  Bitwise OR7/1 -> FiuExp0Bank2/1
  Bitwise AND14/1 -> Bit Shift2/1
  Bitwise AND15/1 -> Bit Shift4/1
  Bus Selector1/3 -> Bitwise AND15/1  "<FaultState>"
  Bus Selector1/4 -> Bitwise AND16/1, Bitwise AND17/1  "<FaultState>"
  Bitwise AND16/1 -> Bit Shift6/1
  Bit Shift6/1 -> Bitwise OR8/3
  Bitwise AND17/1 -> Bit Shift8/1
  Bit Shift8/1 -> Bitwise OR7/1
  Bus Selector1/5 -> Bitwise AND19/1, Bitwise AND18/1  "<FaultState>"
  Bitwise AND18/1 -> Bit Shift11/1
  Bit Shift11/1 -> Bitwise OR7/2
  Bitwise AND19/1 -> Bit Shift12/1
  Bit Shift12/1 -> Bitwise OR9/1
  Bus Selector1/6 -> Bitwise AND20/1  "<FaultState>"
  Bitwise AND20/1 -> Bit Shift13/1
  Bit Shift13/1 -> Bitwise OR9/2
  Bitwise OR9/1 -> FiuExp0Bank3/1
  Bitwise AND21/1 -> Bit Shift14/1
  Bit Shift14/1 -> Bitwise OR9/3
  Bus Selector1/7 -> Bitwise AND22/1, Bitwise AND21/1  "<FaultState>"
  Bitwise AND22/1 -> Bit Shift15/1
  Bit Shift15/1 -> Bitwise OR10/1
  Bitwise OR10/1 -> FiuExp0Bank4/1
  Bitwise AND23/1 -> Bit Shift16/1
  Bit Shift16/1 -> Bitwise OR10/2
  Bus Selector1/8 -> Bitwise AND23/1  "<FaultState>"
  Bitwise OR11/1 -> FiuExp1Bank0/1
  Bitwise AND24/1 -> Bitwise OR11/1
  Bus Selector1/9 -> Bitwise AND24/1  "<FaultState>"
  Bus Selector1/10 -> Bitwise AND26/1, Bitwise AND25/1  "<FaultState>"
  Bitwise AND25/1 -> Bit Shift17/1
  Bit Shift17/1 -> Bitwise OR11/2
  Bitwise OR12/1 -> FiuExp1Bank1/1
  Bitwise AND26/1 -> Bit Shift18/1
  Bit Shift18/1 -> Bitwise OR12/1
  Bit Shift19/1 -> Bitwise OR12/2
  Bitwise AND27/1 -> Bit Shift19/1
  Bus Selector1/11 -> Bitwise AND27/1  "<FaultState>"
  Bitwise AND28/1 -> Bit Shift20/1
  Bit Shift20/1 -> Bitwise OR12/3
  Bus Selector1/12 -> Bitwise AND29/1, Bitwise AND28/1  "<FaultState>"
  Bit Shift21/1 -> FiuExp1Bank2/1
  Bitwise AND29/1 -> Bit Shift21/1

== system speedgoatlib_mscp/Templates/MSCP SC9205 Read Template ==
  Bus Creator : BusCreator  Inputs=12  OutDataTypeStr=Bus: MscpBus_SC9205
      settings: InheritFromInputs=off
  exp0bank{0..4} (5 alike) : slrealtimeethercatlib/EtherCAT PDO Receive  Priority=2  sig_name=Uninitialized Block  sig_offset=144  sig_type=uint8  type_size=8  sig_dim=1  device_id=0  sample_time=0.010000
  exp1bank{0..4} (5 alike) : slrealtimeethercatlib/EtherCAT PDO Receive  Priority=2  sig_name=Uninitialized Block  sig_offset=144  sig_type=uint8  type_size=8  sig_dim=1  device_id=0  sample_time=0.010000
  exp2bank0 : slrealtimeethercatlib/EtherCAT PDO Receive  Priority=2  sig_name=Uninitialized Block  sig_offset=144  sig_type=uint8  type_size=8  sig_dim=1  device_id=0  sample_time=0.010000
  exp2bank1 : slrealtimeethercatlib/EtherCAT PDO Receive  Priority=2  sig_name=Uninitialized Block  sig_offset=144  sig_type=uint8  type_size=8  sig_dim=1  device_id=0  sample_time=0.010000
  Out1 : Outport
  wires:
  Bus Creator/1 -> Out1/1
  exp0bank0/1 -> Bus Creator/1  "Channel_01"
  exp0bank1/1 -> Bus Creator/2  "Channel_02"
  exp0bank2/1 -> Bus Creator/3  "Channel_03"
  exp0bank3/1 -> Bus Creator/4  "Channel_04"
  exp0bank4/1 -> Bus Creator/5  "Channel_05"
  exp1bank0/1 -> Bus Creator/6  "Channel_06"
  exp1bank1/1 -> Bus Creator/7  "Channel_07"
  exp1bank2/1 -> Bus Creator/8  "Channel_08"
  exp1bank3/1 -> Bus Creator/9  "Channel_09"
  exp1bank4/1 -> Bus Creator/10  "Channel_10"
  exp2bank0/1 -> Bus Creator/11  "Channel_11"
  exp2bank1/1 -> Bus Creator/12  "Channel_12"

== system speedgoatlib_mscp/Templates/MSCP SC9205 Write Template ==
  In1 : Inport  OutDataTypeStr=Bus: MscpBus_SC9205
  Bus Selector : BusSelector  OutputSignals=Channel_01,Channel_02,Channel_03,Channel_04,Channel_05,Channel_06,Channel_07,Channel_08,Channel_09,Channel_10,Channel_11,Channel_12
  exp0bank{0..4} (5 alike) : slrealtimeethercatlib/EtherCAT PDO Transmit  Priority=3  sig_name=Uninitialized Block  sig_offset=128  sig_type=uint8  type_size=8  sig_dim=1  device_id=0  sample_time=0.010000
  exp1bank{0..4} (5 alike) : slrealtimeethercatlib/EtherCAT PDO Transmit  Priority=3  sig_name=Uninitialized Block  sig_offset=128  sig_type=uint8  type_size=8  sig_dim=1  device_id=0  sample_time=0.010000
  exp2bank0 : slrealtimeethercatlib/EtherCAT PDO Transmit  Priority=3  sig_name=Uninitialized Block  sig_offset=128  sig_type=uint8  type_size=8  sig_dim=1  device_id=0  sample_time=0.010000
  exp2bank1 : slrealtimeethercatlib/EtherCAT PDO Transmit  Priority=3  sig_name=Uninitialized Block  sig_offset=128  sig_type=uint8  type_size=8  sig_dim=1  device_id=0  sample_time=0.010000
  wires:
  In1/1 -> Bus Selector/1
  Bus Selector/1 -> exp0bank0/1  "<Channel_01>"
  Bus Selector/2 -> exp0bank1/1  "<Channel_02>"
  Bus Selector/3 -> exp0bank2/1  "<Channel_03>"
  Bus Selector/4 -> exp0bank3/1  "<Channel_04>"
  Bus Selector/5 -> exp0bank4/1  "<Channel_05>"
  Bus Selector/6 -> exp1bank0/1  "<Channel_06>"
  Bus Selector/7 -> exp1bank1/1  "<Channel_07>"
  Bus Selector/8 -> exp1bank2/1  "<Channel_08>"
  Bus Selector/9 -> exp1bank3/1  "<Channel_09>"
  Bus Selector/10 -> exp1bank4/1  "<Channel_10>"
  Bus Selector/11 -> exp2bank0/1  "<Channel_11>"
  Bus Selector/12 -> exp2bank1/1  "<Channel_12>"
